simulink model "HW1_pulse"  (R2020b)
settings: Solver=VariableStepAuto  StartTime=0.0  StopTime=10.0  RelTol=1e-3
values from neighbouring files (symbols this model uses):
  delay = delay_set(i)    [HW1.m]
  pulse_amp = pulse_amp_set(i)    [HW1.m]
  pulse_pw = pulse_pw_set(i)    [HW1.m]
settings Model: Creator=ricky  LastModifiedBy=ricky

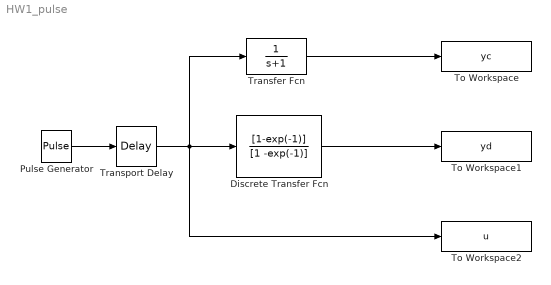
== system HW1_pulse ==
  Discrete Transfer Fcn : DiscreteTransferFcn  Numerator=[1-exp(-1)]  Denominator=[1 -exp(-1)]  SampleTime=1
  Pulse Generator : DiscretePulseGenerator  PulseType=Time based  Amplitude=pulse_amp  Period=10  PulseWidth=pulse_pw  PhaseDelay=1
  To Workspace : ToWorkspace  VariableName=yc  SaveFormat=Timeseries  SampleTime=-1
  To Workspace1 : ToWorkspace  VariableName=yd  SaveFormat=Timeseries  SampleTime=-1
  To Workspace2 : ToWorkspace  VariableName=u  SaveFormat=Timeseries  SampleTime=-1
  Transfer Fcn : TransferFcn  Denominator=[1 1]
  Transport Delay : TransportDelay  DelayTime=delay
  wires:
  Pulse Generator/1 -> Transport Delay/1
  Transfer Fcn/1 -> To Workspace/1
  Discrete Transfer Fcn/1 -> To Workspace1/1
  Transport Delay/1 -> To Workspace2/1, Discrete Transfer Fcn/1, Transfer Fcn/1
